simulink model "run_cartPend_simulink"  (R2015a)
settings: Solver=ode45  StartTime=0.0  StopTime=10.0  RelTol=1e-3
settings Model: Creator=Thomas  LastModifiedBy=Thomas

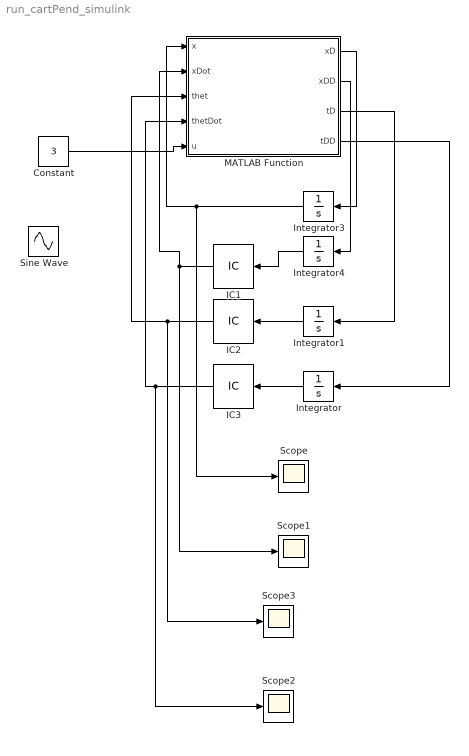
== system run_cartPend_simulink ==
  Constant : Constant  Value=3
  IC1 : InitialCondition  Value=0
  IC2 : InitialCondition  Value=3
  IC3 : InitialCondition  Value=0
  Integrator{,1,3..4} (4 alike) : Integrator
  MATLAB Function : MATLAB Function  TreatAsAtomicUnit=on
  Scope{,1..3} (4 alike) : Scope
      Scope2 settings: SaveName=ScopeData2
      Scope3 settings: SaveName=ScopeData3
  Sine Wave : Sin  SampleTime=0
  wires:
  MATLAB Function/1(xD) -> Integrator3/1
  MATLAB Function/4(tDD) -> Integrator/1
  MATLAB Function/3(tD) -> Integrator1/1
  Integrator4/1 -> IC1/1
  Integrator1/1 -> IC2/1
  Integrator/1 -> IC3/1
  MATLAB Function/2(xDD) -> Integrator4/1
  Integrator3/1 -> MATLAB Function/1(x), Scope/1
  IC1/1 -> MATLAB Function/2(xDot), Scope1/1
  IC3/1 -> Scope2/1, MATLAB Function/4(thetDot)
  IC2/1 -> Scope3/1, MATLAB Function/3(thet)
  Constant/1 -> MATLAB Function/5(u)

== matlab function run_cartPend_simulink/MATLAB Function ==
  data: x input; xDot input; thet input; thetDot input; u input; xD output; xDD output; tD output; tDD output
function [xD,xDD,tD,tDD]  = cartPendSingle( x,xDot,thet,thetDot, u)

mc = 5;
mp = 1;
g = -10;
L = 2;
b = 1;

S = sin( thet );
C = cos( thet );
D = (mc+mp*S.^2);

xD = xDot;
xDD = 1./D .* ( -xDot*b +thetDot.^2.*mp.*L.*S - mp*g*S.*C + u  );
tD =  thetDot;
tDD = 1./D .* ( xDot.*b.*C/L - thetDot.^2.*mp.*S.*C + (mc+mp)*g*S/L + u.*C/L )    ;
